simulink model "pr1"  (Simulink 7.3)
settings: Solver=ode23tb  StartTime=0.0  StopTime=0.2  RelTol=1
libraries: powerlib x14
settings Model: Creator=student  LastModifiedBy=P.R.BHANUTEJA
settings DebuggingCC: FcnCallInpInsideContextMsg=Enable All  StrictBusMsg=ErrorLevel1
settings GRTTargetCC: CombineOutputUpdateFcns=on

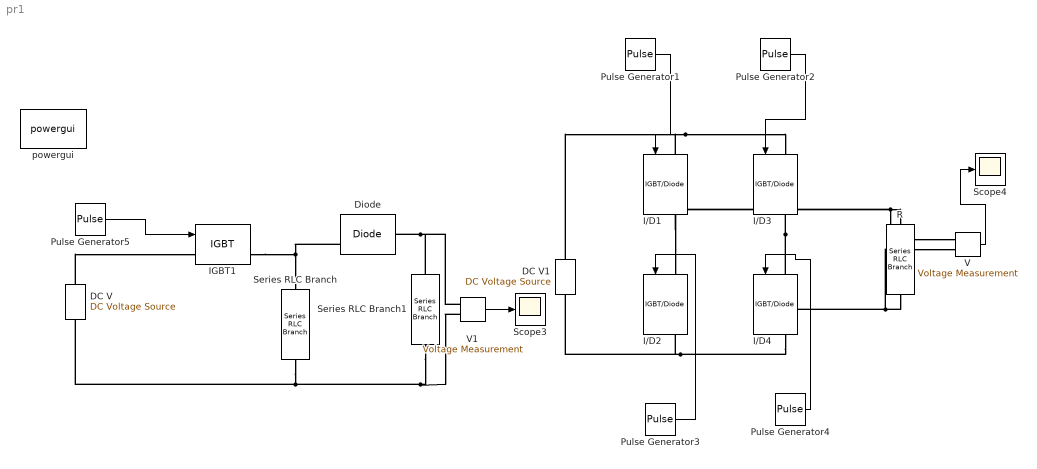
== system pr1 ==
  DC V : powerlib/Electrical Sources/DC Voltage Source  DialogController=POWERSYS.PowerSysDialog  SystemSampleTime=-1  Amplitude=100  Measurements=None
  DC V1 : powerlib/Electrical Sources/DC Voltage Source  DialogController=POWERSYS.PowerSysDialog  SystemSampleTime=-1  Amplitude=100  Measurements=None
  Diode : powerlib/Power Electronics/Diode  DialogController=POWERSYS.PowerSysDialog  SystemSampleTime=-1  Ron=0.001  Lon=0  Vf=0.8  IC=0  UseSnubber=off  Rs=500  Cs=250e-9  Measurements=on
  I/D{1..4} (4 alike) : powerlib/Power Electronics/IGBT//Diode  DialogController=POWERSYS.PowerSysDialog  SystemSampleTime=-1  Ron=1e-3  Rs=1e5  Cs=inf  Measurements=on
  IGBT1 : powerlib/Power Electronics/IGBT  DialogController=POWERSYS.PowerSysDialog  SystemSampleTime=-1  Ron=0.001  Lon=0  Vf=1  Tf=1e-6  Tt=2e-6  IC=0  Rs=1e5  Cs=inf  Measurements=on
  Pulse Generator1 : DiscretePulseGenerator  PulseType=Time based  Amplitude=15  Period=0.02  PulseWidth=50  PhaseDelay=0  SampleTime=1  VectorParams1D=off
  Pulse Generator2 : DiscretePulseGenerator  PulseType=Time based  Amplitude=15  Period=0.02  PulseWidth=50  PhaseDelay=0.01  SampleTime=1  VectorParams1D=off
  Pulse Generator3 : DiscretePulseGenerator  PulseType=Time based  Amplitude=15  Period=0.02  PulseWidth=50  PhaseDelay=0.01  SampleTime=1  VectorParams1D=off
  Pulse Generator4 : DiscretePulseGenerator  PulseType=Time based  Amplitude=15  Period=0.02  PulseWidth=50  PhaseDelay=0  SampleTime=1  VectorParams1D=off
  Pulse Generator5 : DiscretePulseGenerator  PulseType=Time based  TimeSource=Use external signal  Amplitude=15  Period=10  PulseWidth=0.02  PhaseDelay=0  SampleTime=1  VectorParams1D=off
  R : powerlib/Elements/Series RLC Branch  DialogController=POWERSYS.PowerSysDialog  PhysicalDomain=powersysdomain  SubClassName=unknown  LeftPortType=p1  RightPortType=p1  LConnTagsString=__new0  RConnTagsString=__new0  BranchType=R  Resistance=10  Inductance=1e-3  SetiL0=off  InitialCurrent=0  Capacitance=1e-6  Setx0=off  InitialVoltage=0  Measurements=None
  Scope3 : Scope
      settings: TimeRange=0.1  YMin=-5e-07  YMax=5e-07  SaveName=ScopeData2
  Scope4 : Scope
      settings: TimeRange=0.1  YMin=-5e-07  YMax=5e-07  SaveName=ScopeData4
  Series RLC Branch : powerlib/Elements/Series RLC Branch  DialogController=POWERSYS.PowerSysDialog  PhysicalDomain=powersysdomain  SubClassName=unknown  LeftPortType=p1  RightPortType=p1  LConnTagsString=__new0  RConnTagsString=__new0  BranchType=L  Resistance=1  Inductance=100e-6  SetiL0=off  InitialCurrent=0  Capacitance=1e-6  Setx0=off  InitialVoltage=0  Measurements=None
  Series RLC Branch1 : powerlib/Elements/Series RLC Branch  DialogController=POWERSYS.PowerSysDialog  PhysicalDomain=powersysdomain  SubClassName=unknown  LeftPortType=p1  RightPortType=p1  LConnTagsString=__new0  RConnTagsString=__new0  BranchType=C  Resistance=1  Inductance=100e-6  SetiL0=off  InitialCurrent=0  Capacitance=1e-6  Setx0=off  InitialVoltage=0  Measurements=None
  V : powerlib/Measurements/Voltage Measurement  DialogController=POWERSYS.PowerSysDialog  SystemSampleTime=-1  PhasorSimulation=off  OutputType=Complex  PSBequivalent=0
  V1 : powerlib/Measurements/Voltage Measurement  DialogController=POWERSYS.PowerSysDialog  SystemSampleTime=-1  PhasorSimulation=off  OutputType=Complex  PSBequivalent=0
  powergui : powerlib/powergui  Priority=1  SystemSampleTime=-1  SimulationMode=Continuous  SampleTime=50e-6  frequency=60  SPID=off  DisableSnubberDevices=off  DisableRonSwitches=off  DisableVfSwitches=off  SwTol=0  Interpol=off  frequencyindice=0  echomessages=off  HookPort=off  DisplayEquations=off  FunctionMessages=off  EnableUseOfTLC=off  x0status=blocks  RestoreLinks=warning  Frange=[0:2:500]  Ylog=off  Xlog=on  ShowGrid=off  save=off  variable=ZData  ZoomFFT=off  StartTime=0.0  cycles=1  DisplayStyle=1  fundamental=60  FreqAxis=off  MaxFrequency=1000  frequencyindicesteady=1  RmsSteady=1  display=off  Ts=0  methode=off
  wires:
  Pulse Generator1/1 -> I/D1/1
  Pulse Generator2/1 -> I/D3/1
  Pulse Generator4/1 -> I/D4/1
  Pulse Generator3/1 -> I/D2/1
  V/1 -> Scope4/1
  V1/1 -> Scope3/1
  Pulse Generator5/1 -> IGBT1/1
  connections:
  DC V/RConn1 -- IGBT1/LConn1
  IGBT1/RConn1 -- Series RLC Branch/LConn1 -- Diode/RConn1
  V1/LConn2 -- Series RLC Branch1/RConn1 -- Series RLC Branch/RConn1 -- DC V/LConn1
  V1/LConn1 -- Series RLC Branch1/LConn1 -- Diode/LConn1
  I/D1/RConn1 -- I/D2/LConn1 -- R/LConn1 -- V/LConn1
  I/D1/LConn1 -- I/D3/LConn1 -- DC V1/RConn1
  I/D4/RConn1 -- I/D2/RConn1 -- DC V1/LConn1
  R/RConn1 -- I/D4/LConn1 -- I/D3/RConn1 -- V/LConn2
